simulink model "sim4"  (R2024a)
settings: Solver=FixedStepAuto  StartTime=0.0  StopTime=60.0  FixedStep=1e-3  RelTol=1e-3
values from neighbouring files (symbols this model uses):
  zad2 =     [ident_lab2_v08.mat]
libraries: matrix_library x1
settings Model: Creator=alexe  LastModifiedBy=alexe

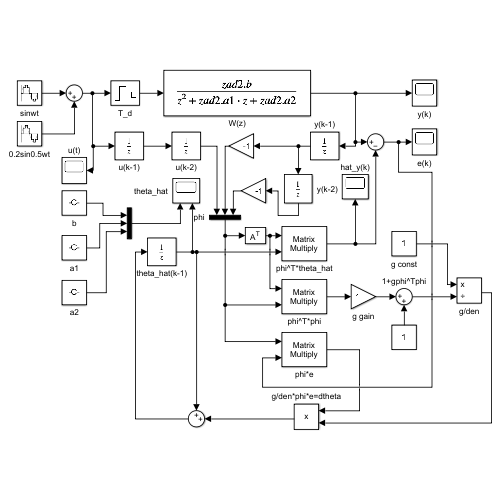
[thumbnail: Simulink's stored preview of the top-level diagram]
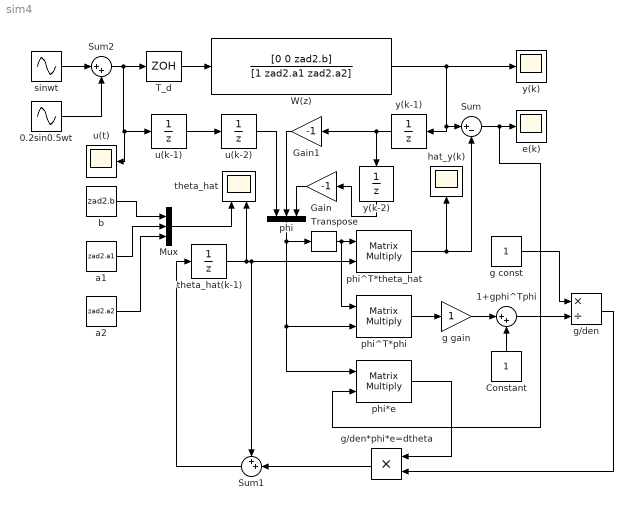
== system sim4 ==
  0.2sin0.5wt : Sin  Amplitude=0.2  Frequency=0.5*zad2.w
  1+gphi^Tphi : Sum  Inputs=|++
  Constant : Constant
  Gain : Gain  Gain=-1
  Gain1 : Gain  Gain=-1
  Mux : Mux  Inputs=3
  Sum : Sum  Inputs=|+-
  Sum1 : Sum  Inputs=++|
  Sum2 : Sum  Inputs=|++
  T_d : ZeroOrderHold  SampleTime=0.1
  Transpose : matrix_library/Transpose
  W(z) : DiscreteTransferFcn  Numerator=[0 0 zad2.b]  Denominator=[1 zad2.a1 zad2.a2]
  a1 : Constant  Value=zad2.a1
  a2 : Constant  Value=zad2.a2
  b : Constant  Value=zad2.b
  e(k) : Scope
  g const : Constant
  g gain : Gain
  g/den : Product  Inputs=*/
  g/den*phi*e=dtheta : Product
  hat_y(k) : Scope
  phi : Mux  Inputs=3
  phi*e : Product  Multiplication=Matrix(*)
  phi^T*phi : Product  Multiplication=Matrix(*)
  phi^T*theta_hat : Product  Multiplication=Matrix(*)
  sinwt : Sin  Frequency=zad2.w
  theta_hat : Scope  NumInputPorts=2
  theta_hat(k-1) : UnitDelay  InitialCondition=[0;0;0];  SampleTime=0.1  HasFrameUpgradeWarning=on
  u(k-1) : UnitDelay  SampleTime=0.1  HasFrameUpgradeWarning=on
  u(k-2) : UnitDelay  SampleTime=0.1  HasFrameUpgradeWarning=on
  u(t) : Scope
  y(k) : Scope
  y(k-1) : UnitDelay  SampleTime=0.1  HasFrameUpgradeWarning=on
  y(k-2) : UnitDelay  SampleTime=0.1  HasFrameUpgradeWarning=on
  wires:
  T_d/1 -> W(z)/1
  W(z)/1 -> y(k-1)/1, Sum/1, y(k)/1
  phi/1 -> Transpose/1, phi*e/1, phi^T*phi/2
  Transpose/1 -> phi^T*phi/1, phi^T*theta_hat/1
  theta_hat(k-1)/1 -> Sum1/1, phi^T*theta_hat/2, theta_hat/2
  phi^T*theta_hat/1 -> Sum/2, hat_y(k)/1
  Sum/1 -> phi*e/2, e(k)/1
  phi^T*phi/1 -> g gain/1
  g gain/1 -> 1+gphi^Tphi/1
  Constant/1 -> 1+gphi^Tphi/2
  g const/1 -> g/den/1
  1+gphi^Tphi/1 -> g/den/2
  phi*e/1 -> g/den*phi*e=dtheta/1
  g/den/1 -> g/den*phi*e=dtheta/2
  g/den*phi*e=dtheta/1 -> Sum1/2
  Sum1/1 -> theta_hat(k-1)/1
  b/1 -> Mux/1
  a1/1 -> Mux/2
  Mux/1 -> theta_hat/1
  u(k-2)/1 -> phi/1
  u(k-1)/1 -> u(k-2)/1
  y(k-1)/1 -> Gain1/1, y(k-2)/1
  Gain/1 -> phi/3
  Gain1/1 -> phi/2
  y(k-2)/1 -> Gain/1
  a2/1 -> Mux/3
  Sum2/1 -> u(t)/1, u(k-1)/1, T_d/1
  sinwt/1 -> Sum2/1
  0.2sin0.5wt/1 -> Sum2/2
